simulink model "district_heating_r2"  (R2018b)
settings: Solver=VariableStepAuto  StartTime=0.0  StopTime=24*3600  RelTol=1e-3
undefined symbols (not defined in the file): DPConstant, DPLinear, DPQuadratic, MassFlow, path_carnot
libraries: carnot x16, Pipe_BiFlow x2, PressureNode x2
settings Model: Creator=drhf  LastModifiedBy=drhf
settings SolverCC: AlgebraicLoopSolver=LineSearch

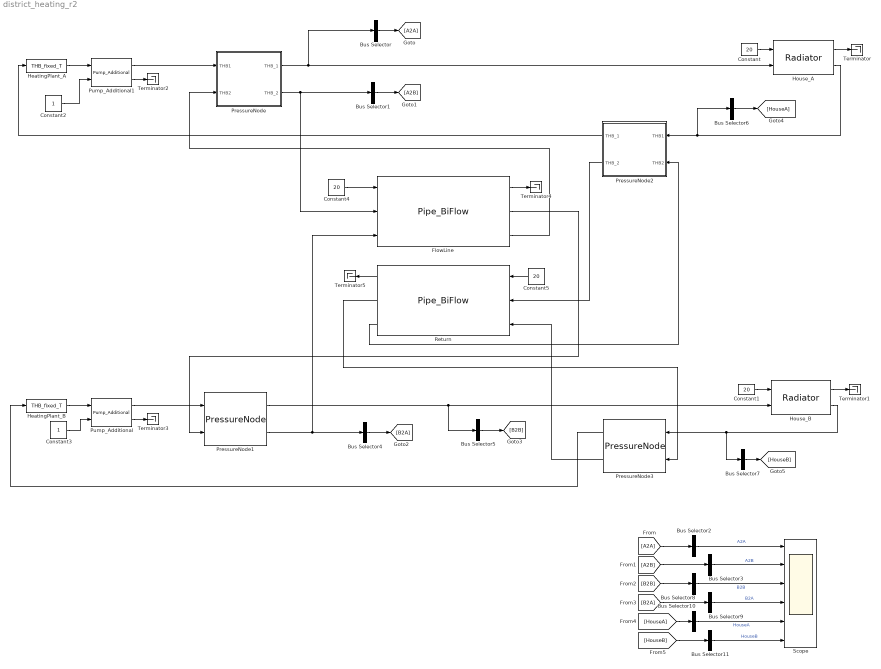
== system district_heating_r2 ==
  Bus Selector{,1,4..7} (6 alike) : BusSelector  OutputSignals=Temperature,MassFlow  OutputAsBus=on
  Bus Selector{2..3,8..11} (6 alike) : BusSelector  OutputSignals=MassFlow  OutputAsBus=on
  Constant{,1,4..5} (4 alike) : Constant  Value=20
  Constant2 : Constant
  Constant3 : Constant
  FlowLine : Pipe_BiFlow/Pipe_BiFlow  t0=20  hgt=254.6479  stgtype=1  tini=[20 20 20 20 20 20 20 20 20 20]  mpts=[1 2 3 4 5 6 7 8 9 10]  PathName=fullfile(path_carnot('libsl'),'Storage','Thermal','Storage_Type_1','parameter_set')  FileName='<user defined>'  userPath=off  userParam=on  uwall=1  ubot=1  utop=1  axcond=1  volume=2  dia=0.1  standing=standing cylinder  nodes=10  mpoints=10  pipe1inlet=1  pipe1outlet=0  pipe1dia=0.1  pipe2inlet=0  pipe2outlet=1  pipe2dia=0.1
  HeatingPlant_A : carnot/Source/Simple/THB_fixed_T  t=70
      settings: SourceProductName=Carnot
  HeatingPlant_B : carnot/Source/Simple/THB_fixed_T  t=60
      settings: SourceProductName=Carnot
  House_A : carnot/Source/Heat_Exchanger/Radiator  pnom=500  dtnom=49.83  expo=1.3  mcap=5*4182  tini=20  lin=10  qua=10
      settings: SourceProductName=Carnot
  House_B : carnot/Source/Heat_Exchanger/Radiator  pnom=500  dtnom=49.83  expo=1.3  mcap=5*4182  tini=20  lin=10  qua=10
      settings: SourceProductName=Carnot
  PressureNode : Subsystem  AncestorBlock=PressureNode/PressureNode
  PressureNode1 : PressureNode/PressureNode  SystemSampleTime=-1
  PressureNode2 : Subsystem  AncestorBlock=PressureNode/PressureNode
  PressureNode3 : PressureNode/PressureNode  SystemSampleTime=-1
  Pump_Additional : carnot/Hydraulics/Pump_Additional  Tini=20  PathName=fullfile(path_carnot('libsl'), 'Hydraulics', 'Pump_Main', 'parameter_set')  FileName='Pump6m.mat'  userPath=off  userParam=off  a0=60000  a1=-43200  a2=0  dia=0.025  UA=1  mcp=4182  e0=50  e1=28.8  e2=-10.368
      settings: SourceProductName=Carnot
  Pump_Additional1 : carnot/Hydraulics/Pump_Additional  Tini=20  PathName=fullfile(path_carnot('libsl'), 'Hydraulics', 'Pump_Main', 'parameter_set')  FileName='Pump6m.mat'  userPath=off  userParam=off  a0=60000  a1=-43200  a2=0  dia=0.025  UA=1  mcp=4182  e0=50  e1=28.8  e2=-10.368
      settings: SourceProductName=Carnot
  Return : Pipe_BiFlow/Pipe_BiFlow  t0=20  hgt=254.6479  stgtype=1  tini=[20 20 20 20 20 20 20 20 20 20]  mpts=[1 2 3 4 5 6 7 8 9 10]  PathName=fullfile(path_carnot('libsl'),'Storage','Thermal','Storage_Type_1','parameter_set')  FileName='<user defined>'  userPath=off  userParam=on  uwall=1  ubot=1  utop=1  axcond=1  volume=2  dia=0.1  standing=standing cylinder  nodes=10  mpoints=10  pipe1inlet=1  pipe1outlet=0  pipe1dia=0.1  pipe2inlet=0  pipe2outlet=1  pipe2dia=0.1
  Scope : Scope  NumInputPorts=6
  Terminator{,1..5} (6 alike) : Terminator
  wires:
  Constant/1 -> House_A/1
  House_A/1 -> Terminator/1
  HeatingPlant_B/1 -> Pump_Additional/1
  HeatingPlant_A/1 -> Pump_Additional1/1
  House_B/1 -> Terminator1/1
  Constant1/1 -> House_B/1
  Pump_Additional1/2 -> Terminator2/1
  Pump_Additional/2 -> Terminator3/1
  Constant2/1 -> Pump_Additional1/2
  Constant3/1 -> Pump_Additional/2
  Constant4/1 -> FlowLine/1
  FlowLine/1 -> Terminator4/1
  Constant5/1 -> Return/1
  House_A/2 -> PressureNode2/1(THB1), Bus Selector6/1
  House_B/2 -> PressureNode3/1, Bus Selector7/1
  Return/1 -> Terminator5/1
  Bus Selector/1 -> [A2A]
  Bus Selector1/1 -> [A2B]
  [A2A] -> Bus Selector2/1
  Bus Selector2/1 -> Scope/1  "A2A"
  [A2B] -> Bus Selector3/1
  Bus Selector3/1 -> Scope/2  "A2B"
  Bus Selector4/1 -> [B2A]
  Bus Selector5/1 -> [B2B]
  Bus Selector6/1 -> [HouseA]
  Bus Selector7/1 -> [HouseB]
  [B2B] -> Bus Selector8/1
  [B2A] -> Bus Selector9/1
  [HouseA] -> Bus Selector10/1
  [HouseB] -> Bus Selector11/1
  Bus Selector8/1 -> Scope/3  "B2B"
  Bus Selector9/1 -> Scope/4  "B2A"
  Bus Selector10/1 -> Scope/5  "HouseA"
  Bus Selector11/1 -> Scope/6  "HouseB"
  PressureNode/2(THB_2) -> FlowLine/2, Bus Selector1/1
  PressureNode/1(THB_1) -> House_A/2, Bus Selector/1
  Pump_Additional1/1 -> PressureNode/1(THB1)
  FlowLine/3 -> PressureNode/2(THB2)
  Pump_Additional/1 -> PressureNode1/1
  FlowLine/2 -> PressureNode1/2
  PressureNode1/2 -> FlowLine/3, Bus Selector4/1
  PressureNode1/1 -> House_B/2, Bus Selector5/1
  Return/3 -> PressureNode2/2(THB2)
  PressureNode2/1(THB_1) -> HeatingPlant_A/1
  PressureNode2/2(THB_2) -> Return/2
  Return/2 -> PressureNode3/2
  PressureNode3/1 -> HeatingPlant_B/1
  PressureNode3/2 -> Return/3

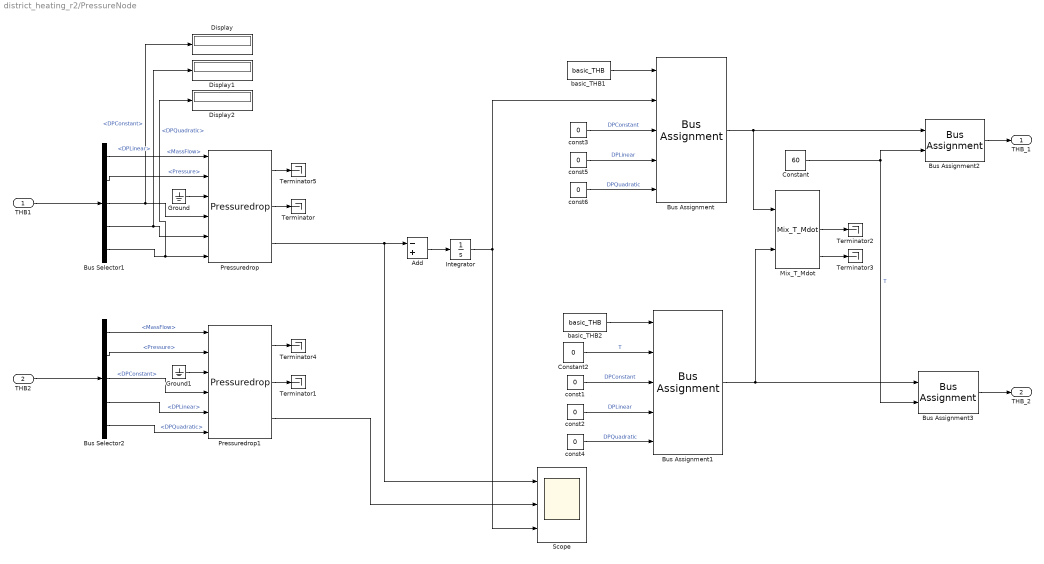
== system district_heating_r2/PressureNode ==
  THB1 : Inport
  THB2 : Inport  Port=2
  Add : Sum  Inputs=-+
  Bus Assignment : BusAssignment  AssignedSignals=MassFlow,DPConstant,DPLinear,DPQuadratic
  Bus Assignment1 : BusAssignment  AssignedSignals=MassFlow,DPConstant,DPLinear,DPQuadratic
  Bus Assignment2 : BusAssignment  AssignedSignals=Temperature
  Bus Assignment3 : BusAssignment  AssignedSignals=Temperature
  Bus Selector1 : BusSelector  OutputSignals=MassFlow,Pressure,DPConstant,DPLinear,DPQuadratic
  Bus Selector2 : BusSelector  OutputSignals=MassFlow,Pressure,DPConstant,DPLinear,DPQuadratic
  Constant : Constant  Value=60
  Constant2 : Constant  Value=0
  Display : Display
  Display1 : Display
  Display2 : Display
  Ground : Ground
  Ground1 : Ground
  Integrator : Integrator  LimitOutput=on  LowerSaturationLimit=0
  Mix_T_Mdot : carnot/Basic/Hydraulics/Mix_T_Mdot  mixcalc=Tmix = (mdot1*T1 + mdot2*T2)/(mdot1+mdot2)
      settings: SourceProductName=Carnot
  Pressuredrop : carnot/Basic/Pressure_Drop/Pressuredrop
      settings: SourceProductName=Carnot
  Pressuredrop1 : carnot/Basic/Pressure_Drop/Pressuredrop
      settings: SourceProductName=Carnot
  Scope : Scope  NumInputPorts=3
  Terminator{,1..5} (6 alike) : Terminator
  basic_THB1 : carnot/Basic/Hydraulics/basic_THB  t=20  mdot=0  p=1e5  ID=Pressure Drop from Massflow  fluid=Water  mix=0  mix2=0  mix3=0  dia=0.02  hgt=0
      settings: SourceProductName=Carnot
  basic_THB2 : carnot/Basic/Hydraulics/basic_THB  t=20  mdot=0  p=1e5  ID=Pressure Drop from Massflow  fluid=Water  mix=0  mix2=0  mix3=0  dia=0.02  hgt=0
      settings: SourceProductName=Carnot
  const{1..6} (6 alike) : Constant  Value=0
  THB_1 : Outport
  THB_2 : Outport  Port=2
  wires:
  const5/1 -> Bus Assignment/4  "DPLinear"
  const6/1 -> Bus Assignment/5  "DPQuadratic"
  THB1/1 -> Bus Selector1/1
  Bus Selector1/1 -> Pressuredrop/1  "<MassFlow>"
  Bus Selector1/2 -> Pressuredrop/2  "<Pressure>"
  Bus Selector1/3 -> Display/1, Pressuredrop/4  "<DPConstant>"
  Bus Selector1/4 -> Display1/1, Pressuredrop/5  "<DPLinear>"
  Bus Selector1/5 -> Display2/1, Pressuredrop/6  "<DPQuadratic>"
  Ground/1 -> Pressuredrop/3
  Pressuredrop/2 -> Terminator/1
  Pressuredrop1/2 -> Terminator1/1
  Ground1/1 -> Pressuredrop1/3
  Bus Selector2/5 -> Pressuredrop1/6  "<DPQuadratic>"
  Bus Selector2/4 -> Pressuredrop1/5  "<DPLinear>"
  Bus Selector2/3 -> Pressuredrop1/4  "<DPConstant>"
  Bus Selector2/2 -> Pressuredrop1/2  "<Pressure>"
  Bus Selector2/1 -> Pressuredrop1/1  "<MassFlow>"
  THB2/1 -> Bus Selector2/1
  basic_THB1/1 -> Bus Assignment/1
  Bus Assignment1/1 -> Bus Assignment3/1, Mix_T_Mdot/2
  Add/1 -> Integrator/1
  Bus Assignment/1 -> Bus Assignment2/1, Mix_T_Mdot/1
  Bus Assignment2/1 -> THB_1/1
  Mix_T_Mdot/2 -> Terminator2/1
  Mix_T_Mdot/3 -> Terminator3/1
  Constant/1 -> Bus Assignment3/2, Bus Assignment2/2  "T"
  Bus Assignment3/1 -> THB_2/1
  const3/1 -> Bus Assignment/3  "DPConstant"
  Pressuredrop/3 -> Add/1, Scope/1
  Pressuredrop1/3 -> Scope/2
  Integrator/1 -> Scope/3, Bus Assignment/2
  Constant2/1 -> Bus Assignment1/2  "T"
  const1/1 -> Bus Assignment1/3  "DPConstant"
  basic_THB2/1 -> Bus Assignment1/1
  const4/1 -> Bus Assignment1/5  "DPQuadratic"
  const2/1 -> Bus Assignment1/4  "DPLinear"
  Pressuredrop/1 -> Terminator5/1
  Pressuredrop1/1 -> Terminator4/1

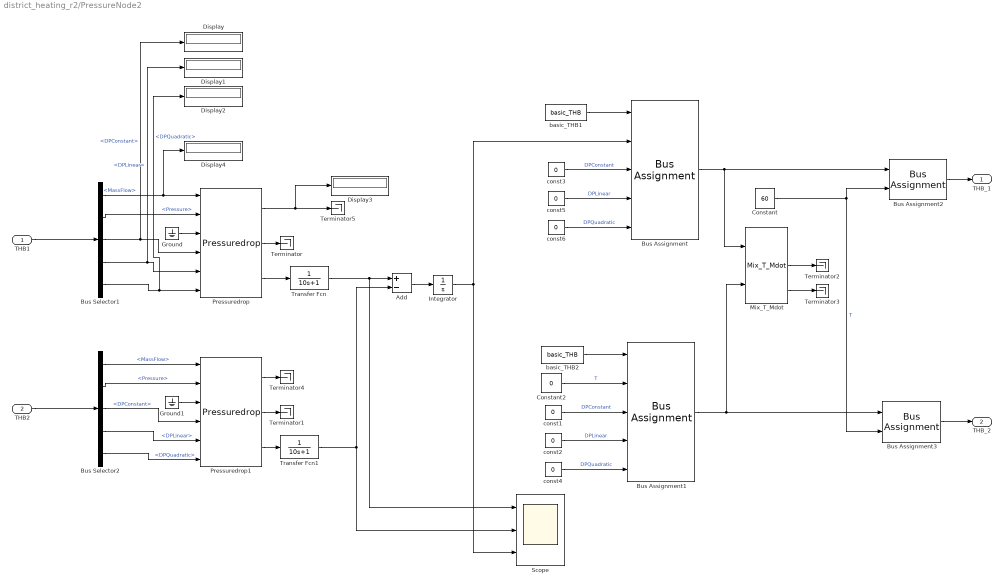
== system district_heating_r2/PressureNode2 ==
  THB1 : Inport
  THB2 : Inport  Port=2
  Add : Sum  Inputs=+-
  Bus Assignment : BusAssignment  AssignedSignals=MassFlow,DPConstant,DPLinear,DPQuadratic
  Bus Assignment1 : BusAssignment  AssignedSignals=MassFlow,DPConstant,DPLinear,DPQuadratic
  Bus Assignment2 : BusAssignment  AssignedSignals=Temperature
  Bus Assignment3 : BusAssignment  AssignedSignals=Temperature
  Bus Selector1 : BusSelector  OutputSignals=MassFlow,Pressure,DPConstant,DPLinear,DPQuadratic
  Bus Selector2 : BusSelector  OutputSignals=MassFlow,Pressure,DPConstant,DPLinear,DPQuadratic
  Constant : Constant  Value=60
  Constant2 : Constant  Value=0
  Display{,1..4} (5 alike) : Display
  Ground : Ground
  Ground1 : Ground
  Integrator : Integrator  LimitOutput=on  LowerSaturationLimit=0
  Mix_T_Mdot : carnot/Basic/Hydraulics/Mix_T_Mdot  mixcalc=Tmix = (mdot1*T1 + mdot2*T2)/(mdot1+mdot2)
      settings: SourceProductName=Carnot
  Pressuredrop : carnot/Basic/Pressure_Drop/Pressuredrop
      settings: SourceProductName=Carnot
  Pressuredrop1 : carnot/Basic/Pressure_Drop/Pressuredrop
      settings: SourceProductName=Carnot
  Scope : Scope  NumInputPorts=3
  Terminator{,1..5} (6 alike) : Terminator
  Transfer Fcn : TransferFcn  Denominator=[10 1]
  Transfer Fcn1 : TransferFcn  Denominator=[10 1]
  basic_THB1 : carnot/Basic/Hydraulics/basic_THB  t=20  mdot=0  p=1e5  ID=Pressure Drop from Massflow  fluid=Water  mix=0  mix2=0  mix3=0  dia=0.02  hgt=0
      settings: SourceProductName=Carnot
  basic_THB2 : carnot/Basic/Hydraulics/basic_THB  t=20  mdot=0  p=1e5  ID=Pressure Drop from Massflow  fluid=Water  mix=0  mix2=0  mix3=0  dia=0.02  hgt=0
      settings: SourceProductName=Carnot
  const{1..6} (6 alike) : Constant  Value=0
  THB_1 : Outport
  THB_2 : Outport  Port=2
  wires:
  Pressuredrop1/3 -> Transfer Fcn1/1
  Pressuredrop1/1 -> Terminator4/1
  Pressuredrop/3 -> Transfer Fcn/1
  Pressuredrop/1 -> Display3/1, Terminator5/1
  const2/1 -> Bus Assignment1/4  "DPLinear"
  const4/1 -> Bus Assignment1/5  "DPQuadratic"
  basic_THB2/1 -> Bus Assignment1/1
  const1/1 -> Bus Assignment1/3  "DPConstant"
  Constant2/1 -> Bus Assignment1/2  "T"
  Integrator/1 -> Bus Assignment/2, Scope/3
  Transfer Fcn1/1 -> Add/2, Scope/2
  Transfer Fcn/1 -> Scope/1, Add/1
  const3/1 -> Bus Assignment/3  "DPConstant"
  Bus Assignment3/1 -> THB_2/1
  Constant/1 -> Bus Assignment2/2, Bus Assignment3/2  "T"
  Mix_T_Mdot/3 -> Terminator3/1
  Mix_T_Mdot/2 -> Terminator2/1
  Bus Assignment2/1 -> THB_1/1
  Bus Assignment/1 -> Mix_T_Mdot/1, Bus Assignment2/1
  Add/1 -> Integrator/1
  Bus Assignment1/1 -> Mix_T_Mdot/2, Bus Assignment3/1
  basic_THB1/1 -> Bus Assignment/1
  THB2/1 -> Bus Selector2/1
  Bus Selector2/1 -> Pressuredrop1/1  "<MassFlow>"
  Bus Selector2/2 -> Pressuredrop1/2  "<Pressure>"
  Bus Selector2/3 -> Pressuredrop1/4  "<DPConstant>"
  Bus Selector2/4 -> Pressuredrop1/5  "<DPLinear>"
  Bus Selector2/5 -> Pressuredrop1/6  "<DPQuadratic>"
  Ground1/1 -> Pressuredrop1/3
  Pressuredrop1/2 -> Terminator1/1
  Pressuredrop/2 -> Terminator/1
  Ground/1 -> Pressuredrop/3
  Bus Selector1/5 -> Pressuredrop/6, Display2/1  "<DPQuadratic>"
  Bus Selector1/4 -> Pressuredrop/5, Display1/1  "<DPLinear>"
  Bus Selector1/3 -> Pressuredrop/4, Display/1  "<DPConstant>"
  Bus Selector1/2 -> Pressuredrop/2  "<Pressure>"
  Bus Selector1/1 -> Display4/1, Pressuredrop/1  "<MassFlow>"
  THB1/1 -> Bus Selector1/1
  const6/1 -> Bus Assignment/5  "DPQuadratic"
  const5/1 -> Bus Assignment/4  "DPLinear"
